simulink model "dummy_system_model"  (R2020a)
settings: Solver=VariableStepAuto  StartTime=0.0  StopTime=10.0  RelTol=1e-3
settings Model: Creator=dhruv  LastModifiedBy=dhruv

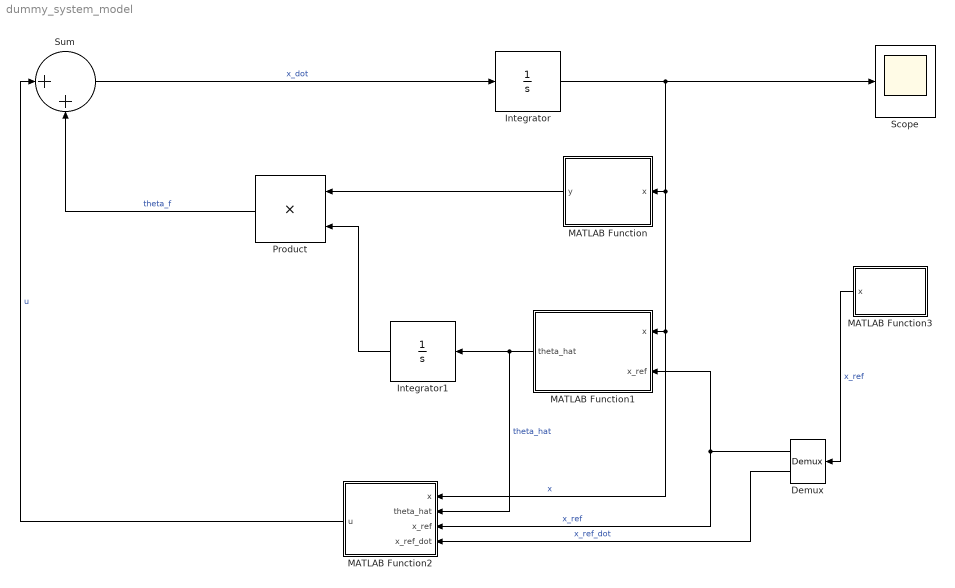
== system dummy_system_model ==
  Demux : Demux  Outputs=2
  Integrator : Integrator
  Integrator1 : Integrator
  MATLAB Function : MATLAB Function  TreatAsAtomicUnit=on
  MATLAB Function1 : MATLAB Function  TreatAsAtomicUnit=on
  MATLAB Function2 : MATLAB Function  TreatAsAtomicUnit=on
  MATLAB Function3 : MATLAB Function  TreatAsAtomicUnit=on
  Product : Product
  Scope : Scope
  Sum : Sum  Inputs=|++
  wires:
  Sum/1 -> Integrator/1  "x_dot"
  Integrator/1 -> MATLAB Function2/1(x), MATLAB Function1/1(x), MATLAB Function/1(x), Scope/1  "x"
  MATLAB Function/1(y) -> Product/1
  Product/1 -> Sum/2  "theta_f"
  MATLAB Function1/1(theta_hat) -> MATLAB Function2/2(theta_hat), Integrator1/1  "theta_hat"
  Integrator1/1 -> Product/2
  MATLAB Function2/1(u) -> Sum/1  "u"
  MATLAB Function3/1(x) -> Demux/1  "x_ref"
  Demux/1 -> MATLAB Function1/2(x_ref), MATLAB Function2/3(x_ref)  "x_ref"
  Demux/2 -> MATLAB Function2/4(x_ref_dot)  "x_ref_dot"

== matlab function dummy_system_model/MATLAB Function1 ==
  data: x input; theta_hat output; x_ref input
function theta_hat = g(x,x_ref)
gamma = 1;

theta_hat = gamma * sin(x) * (x - x_ref);

== matlab function dummy_system_model/MATLAB Function ==
  data: x input; y output
function y = f(x)

y = sin(x);

== matlab function dummy_system_model/MATLAB Function2 ==
  data: x input; u output; theta_hat input; x_ref input; x_ref_dot input
function u = h(x,theta_hat,x_ref,x_ref_dot)
k1 = 1;

u = -theta_hat * sin(x) -x_ref_dot - k1*(x - x_ref);

== matlab function dummy_system_model/MATLAB Function3 ==
  data: x output
function x = fcn()
x(0) = 10; 
x(1) = 0;
